simulink model "verify_Pressure_Drop_StoragePipe_mdl"  (R2016b)
settings: Solver=VariableStepDiscrete  StartTime=0.0  StopTime=10  MaxStep=1  RelTol=1e-3  EnableMultiTasking=on
undefined symbols (not defined in the file or in its folder): DiameterLastPiece, DPConstant, DPLinear, DPQuadratic, Pressure
libraries: carnot x9, simulink x3
settings Model: Creator=drhf  LastModifiedBy=drhf
settings DataIOCC: LimitDataPoints=on  SaveFormat=Array  SignalLoggingSaveFormat=ModelDataLogs
settings OptimizationCC: ExpressionDepthLimit=2147483647  LifeSpan=inf
settings DebuggingCC: UnderspecifiedInitializationDetection=Classic  MergeDetectMultiDrivingBlocksExec=none  SolverPrmCheckMsg=warning  FcnCallInpInsideContextMsg=warning  StateNameClashWarn=warning  SFUnexpectedBacktrackingDiag=warning  SFNoUnconditionalDefaultTransitionDiag=warning  SFExecutionAtInitializationDiag=none
settings HardwareCC: ProdBitPerPointer=32  ProdBitPerSizeT=32  ProdBitPerPtrDiffT=32  ProdLargestAtomicFloat=None  ProdIntDivRoundTo=Undefined  ProdEndianess=Unspecified  ProdWordSize=32  ProdHWDeviceType=32-bit Generic
settings ModelReferenceCC: PropagateSignalLabelsOutOfModel=off
settings GRTTargetCC: TargetLangStandard=C89/C90 (ANSI)  GeneratePreprocessorConditionals=Disable all  CombineOutputUpdateFcns=off  GRTInterface=on
settings ConfigComp: CovMetricSettings=dw  CovHtmlReporting=on  CovSaveCumulativeToWorkspaceVar=on  CovSaveSingleToWorkspaceVar=on  CovExternalEMLEnable=off

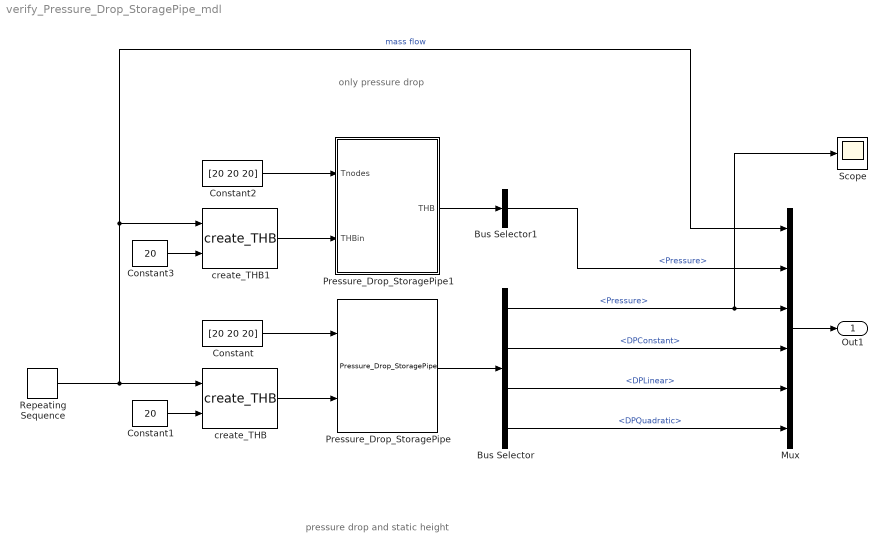
== system verify_Pressure_Drop_StoragePipe_mdl ==
  note: only pressure drop
  note: pressure drop and static height
  Bus Selector : BusSelector  OutputSignals=Pressure,DPConstant,DPLinear,DPQuadratic
  Bus Selector1 : BusSelector  OutputSignals=Pressure
  Constant : Constant  Value=[20 20 20]
  Constant1 : Constant  Value=20
  Constant2 : Constant  Value=[20 20 20]
  Constant3 : Constant  Value=20
  Mux : Mux  Inputs=6
  Pressure_Drop_StoragePipe : carnot/Basic/Pressure_Drop/Pressure_Drop_StoragePipe  dpipe=0.04  dstg=1  hgt=2
  Pressure_Drop_StoragePipe1 : Subsystem  AncestorBlock=carnot/Basic/Pressure_Drop/Pressure_Drop_StoragePipe  mask(Pressure drop pipe connection of a storage){dpipe=0.04, dstg=1, hgt=2}
      mask prompts: dpipe "Diameter of pipe in m"; dstg "Diameter of storage in m"; hgt "Height difference inlet-outlet"
      mask help: Calculates the pressure drop in a pipe connection to a storage respecting the diameter changes and the static height difference. The temperature for the density is taken from the storage nodes.
      mask Help: web(fullfile(path_carnot('help'),'Pressure_Drop_StoragePipe.html'),'-helpbrowser')
      mask TypeOptions dpipe: Pressure_Drop_changeD/dia | Pressure_Drop_decreaseD/dia
      mask TypeOptions dstg: Pressure_Drop_increaseD/dia
      mask TypeOptions hgt: Constant/Value
  Repeating Sequence : simulink/Sources/Repeating Sequence  rep_seq_t=[0 1 9 11]  rep_seq_y=[0 0 1 1]
  Scope : Scope
  create_THB : carnot/Source/Simple/create_THB  p=2e5  fluid=Water  mix=0  mix2=0  mix3=0  dia=0.04  hgt=0  mID=Full Pressure Drop with Static Height
  create_THB1 : carnot/Source/Simple/create_THB  p=2e5  fluid=Water  mix=0  mix2=0  mix3=0  dia=0.04  hgt=0  mID=Pressure Drop from Massflow
  Out1 : Outport
  wires:
  create_THB/1 -> Pressure_Drop_StoragePipe/2
  Pressure_Drop_StoragePipe/1 -> Bus Selector/1
  Constant/1 -> Pressure_Drop_StoragePipe/1
  Constant1/1 -> create_THB/2
  Repeating Sequence/1 -> create_THB1/1, Mux/1, create_THB/1  "mass flow"
  Mux/1 -> Out1/1
  Bus Selector/1 -> Scope/1, Mux/3  "<Pressure>"
  Bus Selector/3 -> Mux/5  "<DPLinear>"
  Bus Selector/4 -> Mux/6  "<DPQuadratic>"
  Bus Selector/2 -> Mux/4  "<DPConstant>"
  Constant2/1 -> Pressure_Drop_StoragePipe1/1(Tnodes)
  create_THB1/1 -> Pressure_Drop_StoragePipe1/2(THBin)
  Pressure_Drop_StoragePipe1/1(THB) -> Bus Selector1/1
  Bus Selector1/1 -> Mux/2  "<Pressure>"
  Constant3/1 -> create_THB1/2

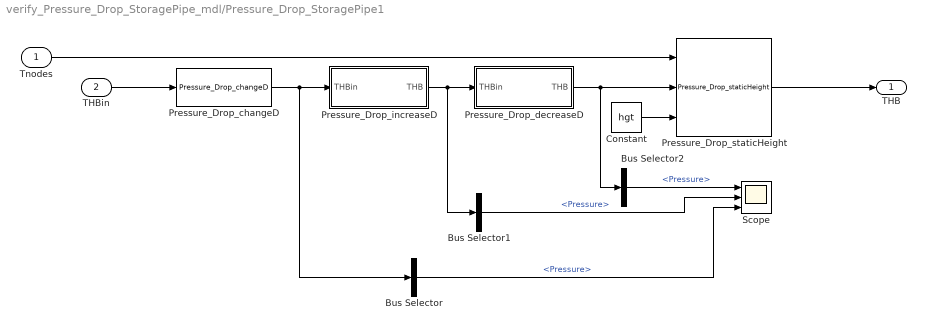
== system verify_Pressure_Drop_StoragePipe_mdl/Pressure_Drop_StoragePipe1 ==
  Tnodes : Inport
  THBin : Inport  Port=2
  Bus Selector : BusSelector  OutputSignals=Pressure
  Bus Selector1 : BusSelector  OutputSignals=Pressure
  Bus Selector2 : BusSelector  OutputSignals=Pressure
  Constant : Constant  Value=hgt
  Pressure_Drop_changeD : carnot/Basic/Pressure_Drop/Pressure_Drop_changeD  dia=dpipe
  Pressure_Drop_decreaseD : Subsystem  AncestorBlock=carnot/Basic/Pressure_Drop/Pressure_Drop_changeD  mask(Pressure Drop Change Diameter){dia=dpipe}
      mask prompts: dia "Diameter in m"
      mask help: Calculates the pressure drop due to a diameter change at the inlet (of a pipe).
      mask Help: web(fullfile(path_carnot('help'),'Pressure_Drop_changeD.html'),'-helpbrowser')
  Pressure_Drop_increaseD : Subsystem  AncestorBlock=carnot/Basic/Pressure_Drop/Pressure_Drop_changeD  mask(Pressure Drop Change Diameter){dia=dstg}
      mask prompts: dia "Diameter in m"
      mask help: Calculates the pressure drop due to a diameter change at the inlet (of a pipe).
      mask Help: web(fullfile(path_carnot('help'),'Pressure_Drop_changeD.html'),'-helpbrowser')
  Pressure_Drop_staticHeight : carnot/Basic/Pressure_Drop/Pressure_Drop_staticHeight
  Scope : Scope  NumInputPorts=3
  THB : Outport
  wires:
  Pressure_Drop_changeD/1 -> Bus Selector/1, Pressure_Drop_increaseD/1(THBin)
  Pressure_Drop_decreaseD/1(THB) -> Bus Selector2/1, Pressure_Drop_staticHeight/2
  Pressure_Drop_staticHeight/1 -> THB/1
  Tnodes/1 -> Pressure_Drop_staticHeight/1
  Pressure_Drop_increaseD/1(THB) -> Bus Selector1/1, Pressure_Drop_decreaseD/1(THBin)
  Constant/1 -> Pressure_Drop_staticHeight/3
  THBin/1 -> Pressure_Drop_changeD/1
  Bus Selector2/1 -> Scope/1  "<Pressure>"
  Bus Selector1/1 -> Scope/2  "<Pressure>"
  Bus Selector/1 -> Scope/3  "<Pressure>"

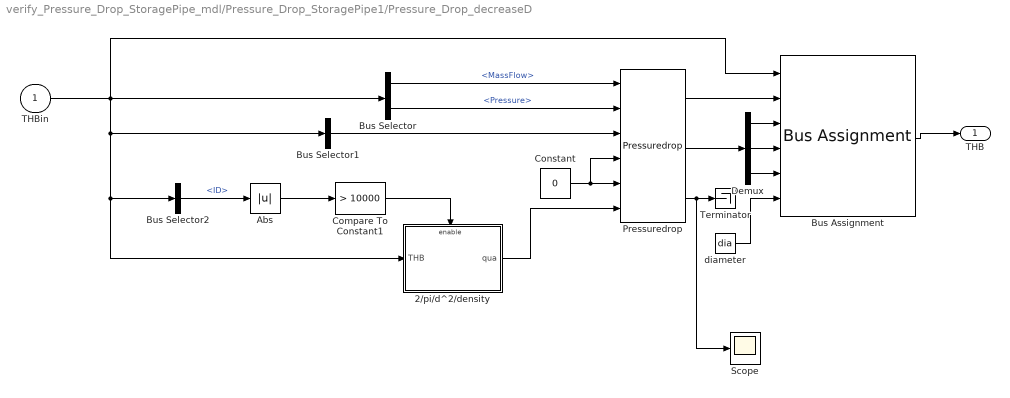
== system verify_Pressure_Drop_StoragePipe_mdl/Pressure_Drop_StoragePipe1/Pressure_Drop_decreaseD ==
  THBin : Inport
  2/pi/d^2/density : Subsystem
  Abs : Abs
  Bus Assignment : BusAssignment  AssignedSignals=Pressure,DPConstant,DPLinear,DPQuadratic,DiameterLastPiece
  Bus Selector : BusSelector  OutputSignals=MassFlow,Pressure
  Bus Selector1 : BusSelector  OutputSignals=DPConstant,DPLinear,DPQuadratic  OutputAsBus=on
  Bus Selector2 : BusSelector  OutputSignals=ID
  Compare To Constant1 : simulink/Logic and Bit Operations/Compare To Constant  relop=>  const=10000  OutDataTypeStr=boolean
  Constant : Constant  Value=0
  Demux : Demux  Outputs=3
  Pressuredrop : carnot/Basic/Pressure_Drop/Pressuredrop
  Scope : Scope
  Terminator : Terminator
  diameter : Constant  Value=dia
  THB : Outport
  wires:
  Pressuredrop/3 -> Scope/1, Terminator/1
  Compare To Constant1/1 -> 2/pi/d^2/density/Enable
  2/pi/d^2/density/1(qua) -> Pressuredrop/6
  Constant/1 -> Pressuredrop/4, Pressuredrop/5
  Bus Selector2/1 -> Abs/1  "<ID>"
  Bus Selector/2 -> Pressuredrop/2  "<Pressure>"
  Bus Selector/1 -> Pressuredrop/1  "<MassFlow>"
  Bus Selector1/1 -> Pressuredrop/3
  Abs/1 -> Compare To Constant1/1
  THBin/1 -> 2/pi/d^2/density/1(THB), Bus Selector2/1, Bus Selector1/1, Bus Selector/1, Bus Assignment/1
  Bus Assignment/1 -> THB/1
  Pressuredrop/1 -> Bus Assignment/2
  Demux/1 -> Bus Assignment/3
  Demux/2 -> Bus Assignment/4
  Demux/3 -> Bus Assignment/5
  Pressuredrop/2 -> Demux/1
  diameter/1 -> Bus Assignment/6

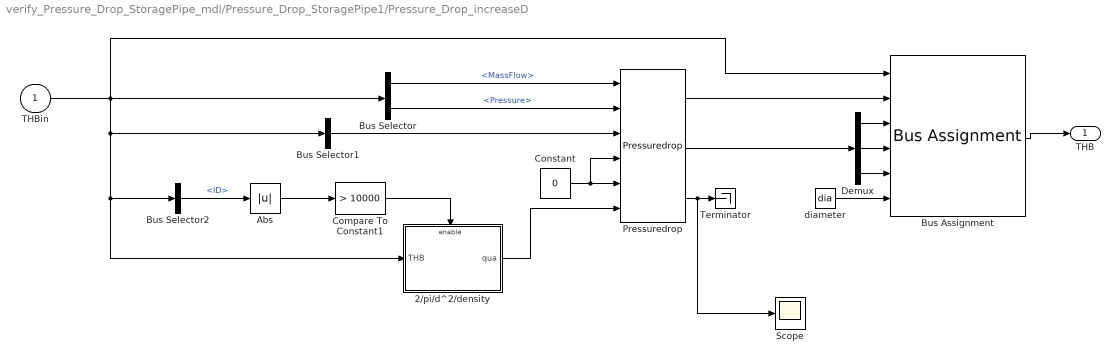
== system verify_Pressure_Drop_StoragePipe_mdl/Pressure_Drop_StoragePipe1/Pressure_Drop_increaseD ==
  THBin : Inport
  2/pi/d^2/density : Subsystem
  Abs : Abs
  Bus Assignment : BusAssignment  AssignedSignals=Pressure,DPConstant,DPLinear,DPQuadratic,DiameterLastPiece
  Bus Selector : BusSelector  OutputSignals=MassFlow,Pressure
  Bus Selector1 : BusSelector  OutputSignals=DPConstant,DPLinear,DPQuadratic  OutputAsBus=on
  Bus Selector2 : BusSelector  OutputSignals=ID
  Compare To Constant1 : simulink/Logic and Bit Operations/Compare To Constant  relop=>  const=10000  OutDataTypeStr=boolean
  Constant : Constant  Value=0
  Demux : Demux  Outputs=3
  Pressuredrop : carnot/Basic/Pressure_Drop/Pressuredrop
  Scope : Scope
  Terminator : Terminator
  diameter : Constant  Value=dia
  THB : Outport
  wires:
  Pressuredrop/3 -> Scope/1, Terminator/1
  Compare To Constant1/1 -> 2/pi/d^2/density/Enable
  2/pi/d^2/density/1(qua) -> Pressuredrop/6
  Constant/1 -> Pressuredrop/4, Pressuredrop/5
  Bus Selector2/1 -> Abs/1  "<ID>"
  Bus Selector/2 -> Pressuredrop/2  "<Pressure>"
  Bus Selector/1 -> Pressuredrop/1  "<MassFlow>"
  Bus Selector1/1 -> Pressuredrop/3
  Abs/1 -> Compare To Constant1/1
  THBin/1 -> 2/pi/d^2/density/1(THB), Bus Selector2/1, Bus Selector1/1, Bus Selector/1, Bus Assignment/1
  Bus Assignment/1 -> THB/1
  Pressuredrop/1 -> Bus Assignment/2
  Demux/1 -> Bus Assignment/3
  Demux/2 -> Bus Assignment/4
  Demux/3 -> Bus Assignment/5
  Pressuredrop/2 -> Demux/1
  diameter/1 -> Bus Assignment/6

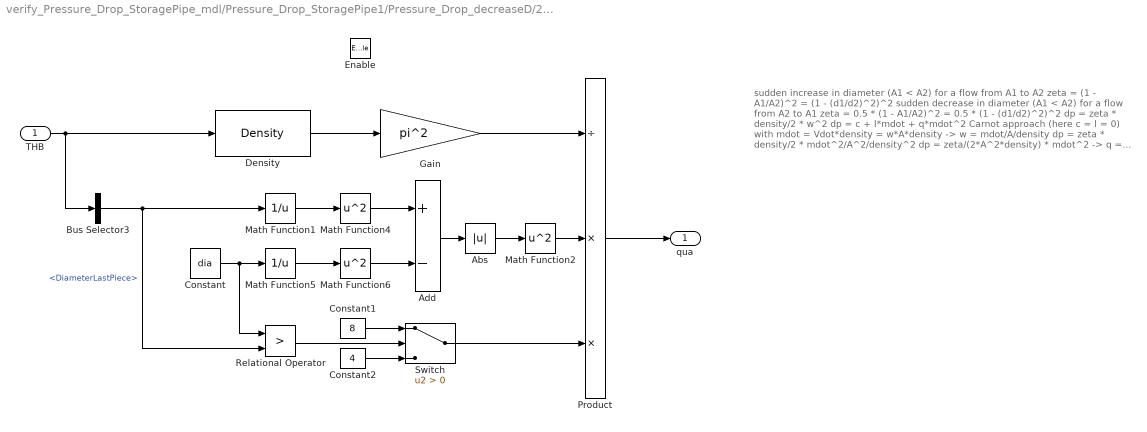
== system verify_Pressure_Drop_StoragePipe_mdl/Pressure_Drop_StoragePipe1/Pressure_Drop_decreaseD/2//pi//d^2//density ==
  note: sudden increase in diameter (A1 < A2)
      |   for a flow from A1 to A2
      |   zeta = (1 - A1/A2)^2 = (1 - (d1/d2)^2)^2
      | sudden decrease in diameter (A1 < A2)
      |   for a flow from A2 to A1
      |   zeta = 0.5 * (1 - A1/A2)^2 = 0.5 * (1 - (d1/d2)^2)^2
      | dp = zeta * density/2 * w^2
      | dp = c + l*mdot + q*mdot^2    Carnot approach (here c = l = 0)
      | with mdot = Vdot*density = w*A*density  -> w = mdot/A/density
      | dp = zeta * density/2 * mdot^2/A^2/density^2
      | dp = zeta/(2*A^2*density) * mdot^2
      | -> q = zeta/(2*A^2*density)
      | diameter increase:
      |   q = (1 - A1/A2)^2/(2*A1^2*density)
      |   q = (1/A1 - 1/A2)^2 / (2*density)
      |   with A = pi/4*d^2
      |   q = 8/density/pi^2 * (1/d1^2 - 1/d2^2)^2
      | diameter decrease:
      |   q = 0.5*(1 - A1/A2)^2/(2*A1^2*density)
      |   q = 0.5*(1/A1 - 1/A2)^2 / (2*density)
      |   with A = pi/4*d^2
      |   q = 4/density/pi^2 * (1/d1^2 - 1/d2^2)^2
  THB : Inport
  Enable : EnablePort
  Abs : Abs
  Add : Sum  Inputs=+-
  Bus Selector3 : BusSelector  OutputSignals=DiameterLastPiece
  Constant : Constant  Value=dia
  Constant1 : Constant  Value=8
  Constant2 : Constant  Value=4
  Density : carnot/Basic/Material_Properties/Density  VariantControl=CarlibClassic  INPUTARGUMENTS=THB  DEBUGLEVEL=DEBUGLEVEL  MAXTOTALWARNINGS=inf  MAXCONSECUTIVEWARNINGS=inf  WRITETOFILE=0  FILENAME='errors.txt'
  Gain : Gain  Gain=pi^2
  Math Function1 : Math  Operator=reciprocal  SaturateOnIntegerOverflow=on
  Math Function2 : Math  Operator=square  SaturateOnIntegerOverflow=on
  Math Function4 : Math  Operator=square  SaturateOnIntegerOverflow=on
  Math Function5 : Math  Operator=reciprocal  SaturateOnIntegerOverflow=on
  Math Function6 : Math  Operator=square  SaturateOnIntegerOverflow=on
  Product : Product  Inputs=/**  RndMeth=Zero
  Relational Operator : RelationalOperator  Operator=>  OutDataTypeStr=boolean  RndMeth=Simplest
  Switch : Switch  Criteria=u2 > Threshold
  qua : Outport
  wires:
  Product/1 -> qua/1
  Gain/1 -> Product/1
  THB/1 -> Density/1, Bus Selector3/1
  Density/1 -> Gain/1
  Bus Selector3/1 -> Relational Operator/2, Math Function1/1  "<DiameterLastPiece>"
  Math Function1/1 -> Math Function4/1
  Math Function5/1 -> Math Function6/1
  Constant/1 -> Relational Operator/1, Math Function5/1
  Relational Operator/1 -> Switch/2
  Constant1/1 -> Switch/1
  Constant2/1 -> Switch/3
  Math Function4/1 -> Add/1
  Math Function6/1 -> Add/2
  Add/1 -> Abs/1
  Abs/1 -> Math Function2/1
  Switch/1 -> Product/3
  Math Function2/1 -> Product/2

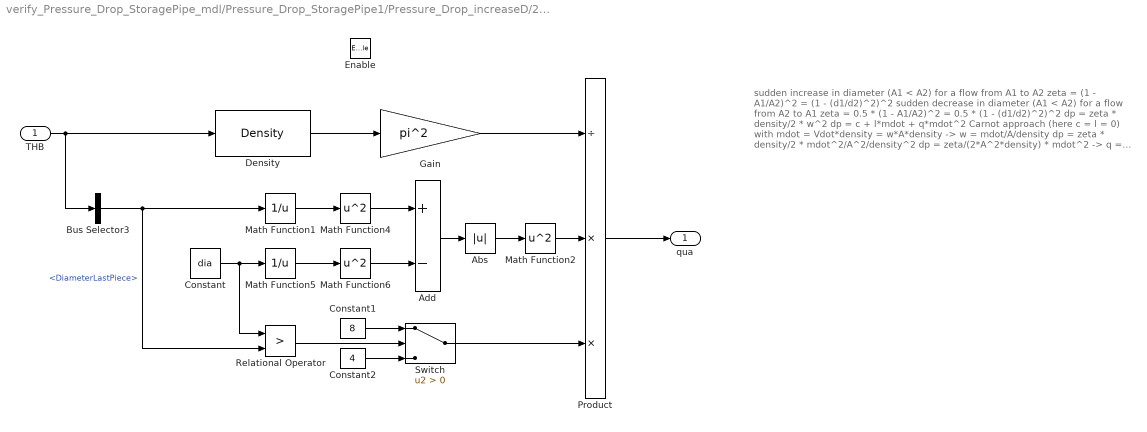
== system verify_Pressure_Drop_StoragePipe_mdl/Pressure_Drop_StoragePipe1/Pressure_Drop_increaseD/2//pi//d^2//density ==
  note: sudden increase in diameter (A1 < A2)
      |   for a flow from A1 to A2
      |   zeta = (1 - A1/A2)^2 = (1 - (d1/d2)^2)^2
      | sudden decrease in diameter (A1 < A2)
      |   for a flow from A2 to A1
      |   zeta = 0.5 * (1 - A1/A2)^2 = 0.5 * (1 - (d1/d2)^2)^2
      | dp = zeta * density/2 * w^2
      | dp = c + l*mdot + q*mdot^2    Carnot approach (here c = l = 0)
      | with mdot = Vdot*density = w*A*density  -> w = mdot/A/density
      | dp = zeta * density/2 * mdot^2/A^2/density^2
      | dp = zeta/(2*A^2*density) * mdot^2
      | -> q = zeta/(2*A^2*density)
      | diameter increase:
      |   q = (1 - A1/A2)^2/(2*A1^2*density)
      |   q = (1/A1 - 1/A2)^2 / (2*density)
      |   with A = pi/4*d^2
      |   q = 8/density/pi^2 * (1/d1^2 - 1/d2^2)^2
      | diameter decrease:
      |   q = 0.5*(1 - A1/A2)^2/(2*A1^2*density)
      |   q = 0.5*(1/A1 - 1/A2)^2 / (2*density)
      |   with A = pi/4*d^2
      |   q = 4/density/pi^2 * (1/d1^2 - 1/d2^2)^2
  THB : Inport
  Enable : EnablePort
  Abs : Abs
  Add : Sum  Inputs=+-
  Bus Selector3 : BusSelector  OutputSignals=DiameterLastPiece
  Constant : Constant  Value=dia
  Constant1 : Constant  Value=8
  Constant2 : Constant  Value=4
  Density : carnot/Basic/Material_Properties/Density  VariantControl=CarlibClassic  INPUTARGUMENTS=THB  DEBUGLEVEL=DEBUGLEVEL  MAXTOTALWARNINGS=inf  MAXCONSECUTIVEWARNINGS=inf  WRITETOFILE=0  FILENAME='errors.txt'
  Gain : Gain  Gain=pi^2
  Math Function1 : Math  Operator=reciprocal  SaturateOnIntegerOverflow=on
  Math Function2 : Math  Operator=square  SaturateOnIntegerOverflow=on
  Math Function4 : Math  Operator=square  SaturateOnIntegerOverflow=on
  Math Function5 : Math  Operator=reciprocal  SaturateOnIntegerOverflow=on
  Math Function6 : Math  Operator=square  SaturateOnIntegerOverflow=on
  Product : Product  Inputs=/**  RndMeth=Zero
  Relational Operator : RelationalOperator  Operator=>  OutDataTypeStr=boolean  RndMeth=Simplest
  Switch : Switch  Criteria=u2 > Threshold
  qua : Outport
  wires:
  Product/1 -> qua/1
  Gain/1 -> Product/1
  THB/1 -> Density/1, Bus Selector3/1
  Density/1 -> Gain/1
  Bus Selector3/1 -> Relational Operator/2, Math Function1/1  "<DiameterLastPiece>"
  Math Function1/1 -> Math Function4/1
  Math Function5/1 -> Math Function6/1
  Constant/1 -> Relational Operator/1, Math Function5/1
  Relational Operator/1 -> Switch/2
  Constant1/1 -> Switch/1
  Constant2/1 -> Switch/3
  Math Function4/1 -> Add/1
  Math Function6/1 -> Add/2
  Add/1 -> Abs/1
  Abs/1 -> Math Function2/1
  Switch/1 -> Product/3
  Math Function2/1 -> Product/2
